simulink model "Question_5"  (R2024b)
settings: Solver=VariableStepAuto  StartTime=0.0  StopTime=34  RelTol=1e-3
model workspace (MAT data in the model file):
  Voltage = 1
settings Model: Creator=Sagar  LastModifiedBy=Sagar
settings DataIOCC: InspectSignalLogs=on

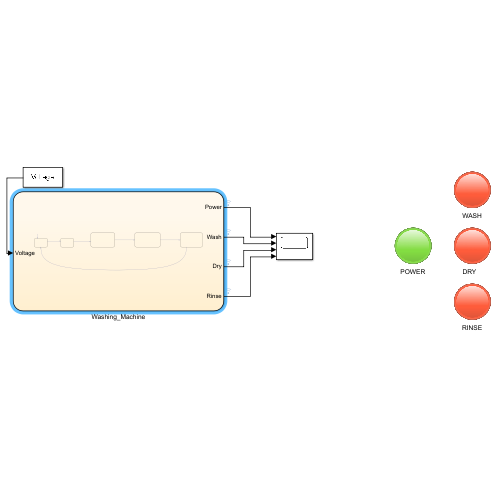
[thumbnail: Simulink's stored preview of the top-level diagram]
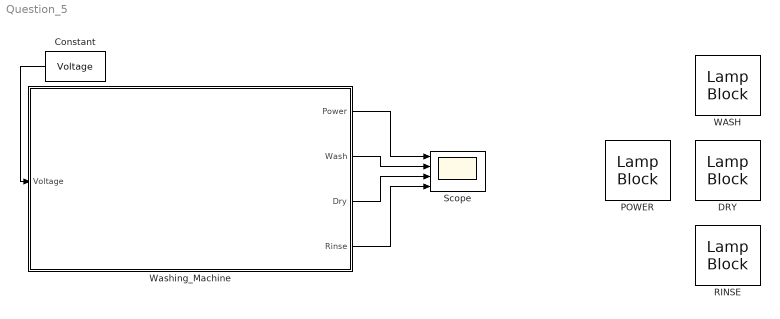
== system Question_5 ==
  Constant : Constant  Value=Voltage
  "DRY   " : LampBlock  LabelPosition=Hide
  POWER : LampBlock  LabelPosition=Hide
  RINSE : LampBlock  LabelPosition=Hide
  Scope : Scope  NumInputPorts=4
  WASH : LampBlock  LabelPosition=Hide
  Washing_Machine : Stateflow chart  TreatAsAtomicUnit=on
  wires:
  Constant/1 -> Washing_Machine/1(Voltage)
  Washing_Machine/1(Power) -> Scope/1
  Washing_Machine/2(Wash) -> Scope/2
  Washing_Machine/3(Dry) -> Scope/3
  Washing_Machine/4(Rinse) -> Scope/4

== stateflow chart Question_5/Washing_Machine ==
  state Washing
    entry:
    after(20,sec)
  state Rinsing
    entry:
    after(10,sec)
  state Drying
    entry:
    after(3,sec)
  state OFF
    exit: stop;
  state ON
    after(1,sec)
  (default) -> OFF
  Washing -> Rinsing : {Wash=0;Rinse = 1}
  Rinsing -> Drying : {Rinse=0;Dry=1}
  OFF -> ON : {Power=1}
  ON -> Washing : {Wash=1}
  Drying -> OFF : {Power=0;Dry=0}
  data: Voltage input; Power output; Wash output; Dry output; Rinse output
